simulink model "simulink_01"  (R2017b)
settings: Solver=VariableStepAuto  StartTime=0.0  StopTime=10  RelTol=1e-3
settings Model: Creator=hp  LastModifiedBy=hp

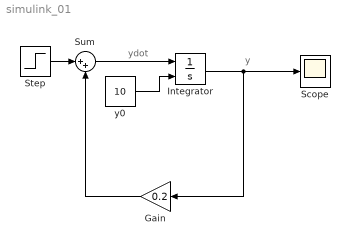
== system simulink_01 ==
  note: y
  note: ydot
  Gain : Gain  Gain=0.2
  Integrator : Integrator  InitialConditionSource=external  InitialCondition=50  ContinuousStateAttributes='y0'
  Scope : Scope
  Step : Step  After=0  SampleTime=0
  Sum : Sum  Inputs=|++
  y0 : Constant  Value=10
  wires:
  Integrator/1 -> Scope/1, Gain/1
  Gain/1 -> Sum/2
  Step/1 -> Sum/1
  Sum/1 -> Integrator/1
  y0/1 -> Integrator/2
